simulink model "Go_Kart_Model_2018"  (R2019a)
settings: Solver=VariableStepAuto  StartTime=0.0  StopTime=2  RelTol=1e-3
model workspace (MAT data in the model file):
  Air_Resistance = Simulink.Parameter
  Air_Resistance.Value = 0.26903
  Air_Resistance.DataType = 'auto'
  Air_Resistance.DocUnits = 'kg/m'
  Air_Resistance.Dimensions = [1 1]
  Gear_Ratio = Simulink.Parameter
  Gear_Ratio.Value = 12.75
  Gear_Ratio.DataType = 'auto'
  Gear_Ratio.Dimensions = [1 1]
  Mass = Simulink.Parameter
  Mass.Value = 200
  Mass.DataType = 'auto'
  Mass.DocUnits = 'kg'
  Mass.Dimensions = [1 1]
  Num_Motors = Simulink.Parameter
  Num_Motors.Value = 6
  Num_Motors.DataType = 'auto'
  Num_Motors.Dimensions = [1 1]
  Tire_Radius = Simulink.Parameter
  Tire_Radius.Value = 0.2286
  Tire_Radius.DataType = 'auto'
  Tire_Radius.DocUnits = 'm'
  Tire_Radius.Dimensions = [1 1]
settings Model: OrderedModelArguments=off  Creator=hanso  LastModifiedBy=chanson
settings DataIOCC: ReturnWorkspaceOutputs=off
settings DebuggingCC: ArithmeticOperatorsInVariantConditions=warning

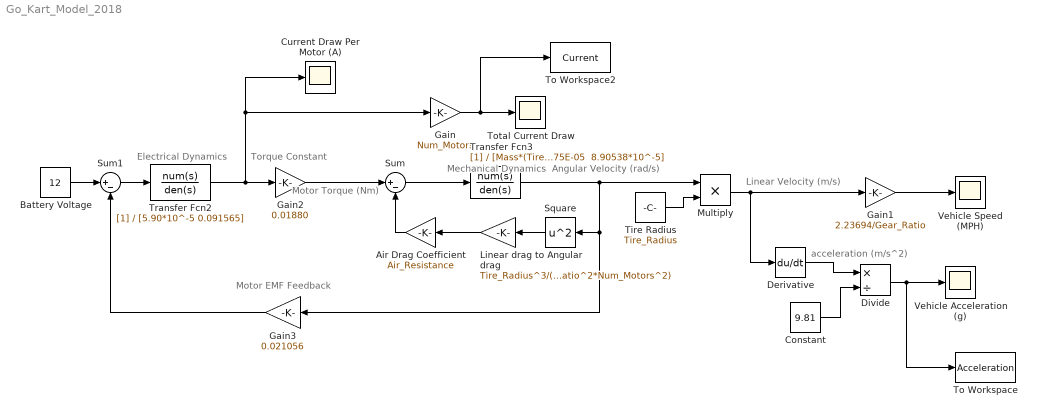
== system Go_Kart_Model_2018 ==
  note: Angular Velocity (rad/s)
  note: acceleration (m/s^2)
  note: Linear Velocity (m/s)
  note: Torque Constant
  note: Electrical Dynamics
  note: Mechanical Dynamics
  note: Motor Torque (Nm)
  note: Motor EMF Feedback
  Air Drag Coefficient : Gain  Gain=Air_Resistance
  Battery Voltage : Constant  Value=12
  Constant : Constant  Value=9.81
  Current Draw Per Motor (A) : Scope
  Derivative : Derivative
  Divide : Product  Inputs=*/
  Gain : Gain  Gain=Num_Motors
  Gain1 : Gain  Gain=2.23694/Gear_Ratio
  Gain2 : Gain  Gain=0.01880
  Gain3 : Gain  Gain=0.021056
  Linear drag to Angular drag : Gain  Gain=Tire_Radius^3/(Gear_Ratio^2*Num_Motors^2)
  Multiply : Product
  Square : Math  Operator=square  SaturateOnIntegerOverflow=on
  Sum : Sum  Inputs=|+-
  Sum1 : Sum  Inputs=|+-
  Tire Radius : Constant  Value=Tire_Radius
  To Workspace : ToWorkspace  VariableName=Acceleration  SaveFormat=Timeseries  SampleTime=-1
  To Workspace2 : ToWorkspace  VariableName=Current  SaveFormat=Timeseries  SampleTime=-1
  Total Current Draw : Scope
  Transfer Fcn2 : TransferFcn  Denominator=[5.90*10^-5 0.091565]
  Transfer Fcn3 : TransferFcn  Denominator=|
      | [Mass*(Tire_Radius)^2/(Gear_Ratio^2*Num_Motors^2)+7.75E-05
      | 
      |  8.90538*10^-5]
  Vehicle Acceleration (g) : Scope
  Vehicle Speed (MPH) : Scope
  wires:
  Gain3/1 -> Sum1/2
  Sum1/1 -> Transfer Fcn2/1
  Tire Radius/1 -> Multiply/2
  Multiply/1 -> Derivative/1, Gain1/1
  Gain1/1 -> Vehicle Speed (MPH)/1
  Battery Voltage/1 -> Sum1/1
  Transfer Fcn2/1 -> Gain/1, Current Draw Per Motor (A)/1, Gain2/1
  Gain2/1 -> Sum/1
  Sum/1 -> Transfer Fcn3/1
  Transfer Fcn3/1 -> Gain3/1, Square/1, Multiply/1
  Square/1 -> Linear drag to Angular drag/1
  Air Drag Coefficient/1 -> Sum/2
  Linear drag to Angular drag/1 -> Air Drag Coefficient/1
  Derivative/1 -> Divide/1
  Constant/1 -> Divide/2
  Divide/1 -> To Workspace/1, Vehicle Acceleration (g)/1
  Gain/1 -> To Workspace2/1, Total Current Draw/1
